simulink model "costas_baseband"  (Simulink 5.0)
settings: Solver=ode45  StartTime=0.0  StopTime=2  RelTol=1e-3
libraries: dsparch4 x3, commcontsrc2 x2, dspsigops x2, commdigbbndpm2 x1, commrflib2 x1, commrandsrc2 x1
settings Model: LastModifiedBy=Daiming Qu

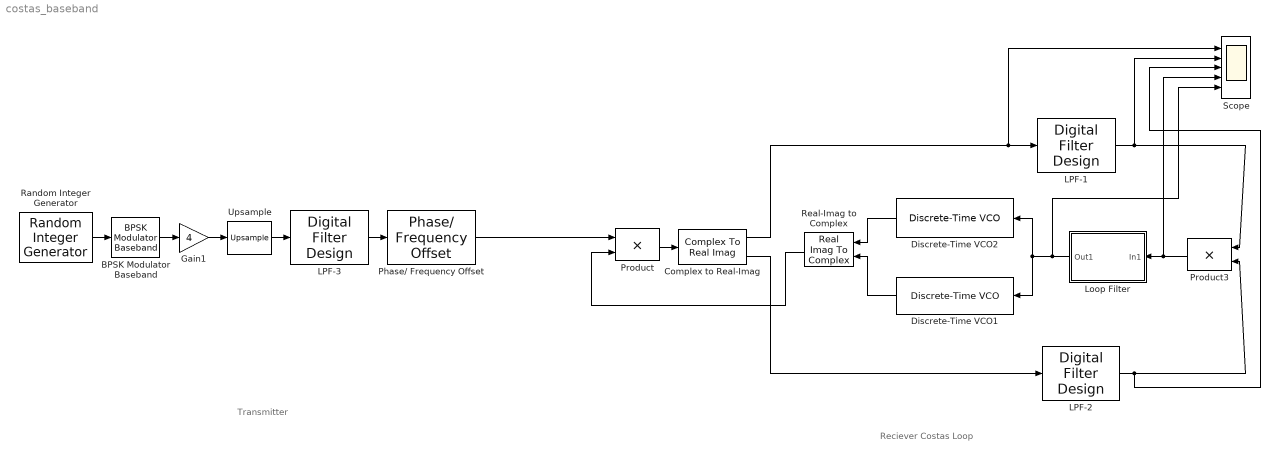
== system costas_baseband ==
  note: Transmitter
  note: Reciever
      | Costas Loop
  BPSK Modulator Baseband : commdigbbndpm2/BPSK Modulator Baseband  Ph=0  numSamp=1
  Complex to Real-Imag : ComplexToRealImag
  Discrete-Time VCO1 : commcontsrc2/Discrete-Time VCO  Orientation=left  Ac=1  Fc=0  Kc=1  Ph=pi/2  ts=1/1000
  Discrete-Time VCO2 : commcontsrc2/Discrete-Time VCO  Orientation=left  Ac=1  Fc=0  Kc=1  Ph=0  ts=1/1000
  Gain1 : Gain  Gain=4  SaturateOnIntegerOverflow=on
  LPF-1 : dsparch4/Digital Filter Design
  LPF-2 : dsparch4/Digital Filter Design
  LPF-3 : dsparch4/Digital Filter Design
  Loop Filter : Subsystem  Orientation=left
  Phase/ Frequency Offset : commrflib2/Phase// Frequency Offset  freqOffset=1  phaseOffset=0
  Product : Product  SaturateOnIntegerOverflow=on
  Product3 : Product  Orientation=left  SaturateOnIntegerOverflow=on
  Random Integer Generator : commrandsrc2/Random Integer Generator  mul=2  seed=37  Ts=1/250  frameBased=off  sampPerFrame=1  orient=off
  Real-Imag to Complex : RealImagToComplex  Orientation=left
  Scope : Scope  NumInputPorts=5
      settings: YMin=-1.5~-5~-1~0~0  YMax=1.5~5~1~2~2
  Upsample : dspsigops/Upsample  N=4  phase=0  ic=0  mode=Maintain input frame size
  wires:
  Discrete-Time VCO2/1 -> Real-Imag to Complex/1
  Complex to Real-Imag/1 -> Scope/1, LPF-1/1
  LPF-1/1 -> Scope/2, Product3/1
  Random Integer Generator/1 -> BPSK Modulator Baseband/1
  Discrete-Time VCO1/1 -> Real-Imag to Complex/2
  BPSK Modulator Baseband/1 -> Gain1/1
  Upsample/1 -> LPF-3/1
  LPF-2/1 -> Product3/2, Scope/3
  Gain1/1 -> Upsample/1
  LPF-3/1 -> Phase/ Frequency Offset/1
  Phase/ Frequency Offset/1 -> Product/1
  Real-Imag to Complex/1 -> Product/2
  Product/1 -> Complex to Real-Imag/1
  Complex to Real-Imag/2 -> LPF-2/1
  Loop Filter/1(Out1) -> Discrete-Time VCO2/1, Discrete-Time VCO1/1, Scope/5
  Product3/1 -> Loop Filter/1(In1), Scope/4

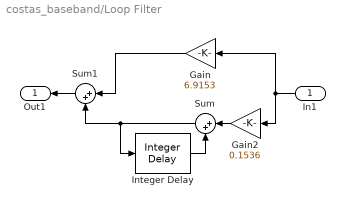
== system costas_baseband/Loop Filter ==
  In1 : Inport  Orientation=left
  Gain : Gain  Orientation=left  Gain=6.9153  SaturateOnIntegerOverflow=on
  Gain2 : Gain  Orientation=left  Gain=0.1536  SaturateOnIntegerOverflow=on
  Integer Delay : dspsigops/Integer Delay  delay=1  ic=0  reset_popup=None
  Sum : Sum  Orientation=left  Inputs=|++  SaturateOnIntegerOverflow=on
  Sum1 : Sum  Orientation=left  Inputs=|++  SaturateOnIntegerOverflow=on
  Out1 : Outport  Orientation=left
  wires:
  Gain2/1 -> Sum/1
  Gain/1 -> Sum1/1
  Sum/1 -> Integer Delay/1, Sum1/2
  Integer Delay/1 -> Sum/2
  In1/1 -> Gain2/1, Gain/1
  Sum1/1 -> Out1/1
